simulink model "USRPEmetteur"  (R2017b)
settings: Solver=VariableStepAuto  StartTime=0.0  StopTime=10.0  RelTol=1e-3
libraries: commrandsrc3 x1, commdigbbndpm3 x1, commfilt2 x1, commsdrhw_v2 x1
settings Model: Creator=Clementg20  LastModifiedBy=Clementg20

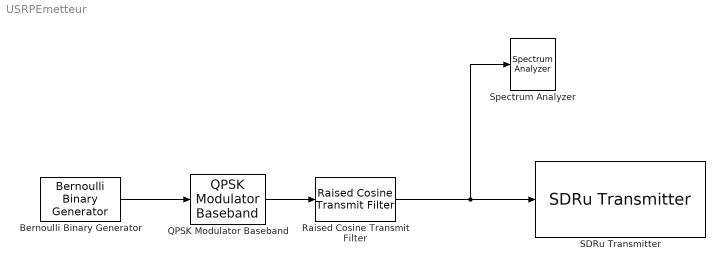
== system USRPEmetteur ==
  Bernoulli Binary Generator : commrandsrc3/Bernoulli Binary Generator  ProbabilityOfZero=0.5  SeedSource=Auto  Seed=0  SampleTime=0.5e-6  SamplesPerFrame=2  OutputDataType=double  SimulateUsing=Interpreted execution
  QPSK Modulator Baseband : commdigbbndpm3/QPSK Modulator Baseband  InType=Bit  Enc=Gray  Ph=pi/4  outDtype=double  outWordLen=16  outUDDataType=sfix(16)  outFracLenMode=Best precision  outFracLen=15  outDataTypeStr=double  outLastDataTypeStr=double
  Raised Cosine Transmit Filter : commfilt2/Raised Cosine Transmit Filter  filtType=Square root  R=0.2  filtSpan=12  N=4  filterGain=1  InputProcessing=Columns as channels (frame based)  RateOptions=Allow multirate processing  framing=Mute  checkCoeff=off  variableName=rcTxFilt  checkGain=Normalized  sampMode=Mute  saveAsFlag=0  currentFiltSpan=12  D=(12)/2  launchFVT=on  roundingMode=Floor  overflowMode=off  coeffDataTypeStr=Inherit: Same word length as input  coeffMin=[]  coeffMax=[]  coeffLastDataTypeStr=Inherit: Same word length as input  outputDataTypeStr=Inherit: Same as accumulator  outputMin=[]  outputMax=[]  outputLastDataTypeStr=Inherit: Same as accumulator
  SDRu Transmitter : commsdrhw_v2/SDRu Transmitter  SourceLibraryInfo="This block requires <a href=\"http://www.mathworks.com/hardware-support/usrp.html\">Communications System Toolbox Support Package for USRP Radio</a>"  rxtx=tx  platform=B210  USRP2_IP='192.168.10.2'  USRP_IP_X300='192.168.10.2'  USRP_IP_X310='192.168.10.2'  USRP_serialNumB200=''  USRP_serialNumB210='30CEE99'  ChannelMapping=1  centerFrequency=2.45e9  centerFrequencySrc=Dialog  loOffset=0  loOffsetSrc=Dialog  PPSSource=Internal  clockSource=Internal  masterClkRateB200=32e6  masterClkRateB210=2.0480e9  masterClkRateX300=200e6  masterClkRateX310=200e6  masterClkRateParam=61440000  gain=200  gainSrc=Dialog  decimInterp=512  decimInterpSrc=Dialog  TransportDataType=int16  USRP2_IP_NUM=[51 48 67 69 69 57 57]  frameLength=362  outputDatatype=Same as transport data type  overrunUnderrunPort=off  sampleTime=1  dboardInfo=|  HOST_DATA_PORT=30000  HOST_CONTROL_PORT=30001  USRP2_DATA_PORT=32769  USRP2_CONTROL_PORT=32768  bufferMode=Continuous streaming  EnableBurstMode=off  NumFramesInBurst=100  USRP_ID='30CEE99'
      | dbid: 0
      |           dbName: 'no db found'
      |          freqMin: 0
      |          freqMax: 0
      |          gainMin: 0
      |          gainMax: 0
      |     gainStepSize: 0
      settings: SourceProductName=Communications System Toolbox Support Package for USRP(R) Radio  SourceProductBaseCode=USRP
  Spectrum Analyzer : SpectrumAnalyzer
  wires:
  Bernoulli Binary Generator/1 -> QPSK Modulator Baseband/1
  Raised Cosine Transmit Filter/1 -> Spectrum Analyzer/1, SDRu Transmitter/1
  QPSK Modulator Baseband/1 -> Raised Cosine Transmit Filter/1
